simulink model "single_ph_controlled_rectifier_inductive_load"  (R2018a)
settings: Solver=ode23tb  StartTime=0  StopTime=2  MaxStep=1e-6  RelTol=1e-5
libraries: powerlib x10
settings Model: Creator=pranjal  LastModifiedBy=pranjal
settings HardwareCC: ProdBitPerLong=64  ProdHWDeviceType=AMD->x86-64 (Linux 64)

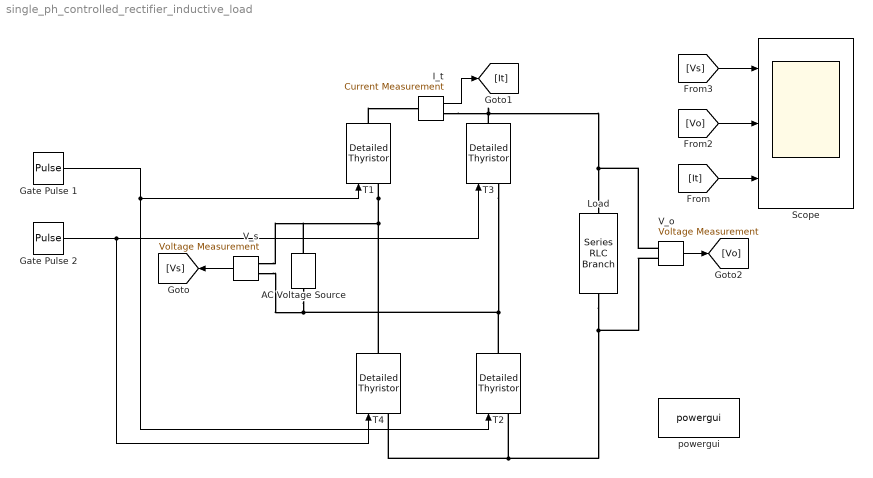
== system single_ph_controlled_rectifier_inductive_load ==
  AC Voltage Source : powerlib/Electrical Sources/AC Voltage Source  Amplitude=230*1.414  Phase=0  Frequency=50  SampleTime=0  Measurements=Voltage  BusType=swing  Pref=10e3  Qref=0  Qmin=-inf  Qmax=+inf
  Gate Pulse 1 : DiscretePulseGenerator  PulseType=Time based  Period=20e-3  PulseWidth=5  PhaseDelay=(30/360)*20e-3
  Gate Pulse 2 : DiscretePulseGenerator  PulseType=Time based  Period=20e-3  PulseWidth=5  PhaseDelay=((180+30)/360)*20e-3
  I_t : powerlib/Measurements/Current Measurement  PhasorSimulation=off  OutputType=Complex  PSBequivalent=0
  Load : powerlib/Elements/Series RLC Branch  LConnTagsString=__new0  RConnTagsString=__new0  BranchType=RL  Resistance=20  Inductance=5  SetiL0=off  InitialCurrent=0  Capacitance=1e-6  Setx0=off  InitialVoltage=0  Measurements=None
  Scope : Scope  NumInputPorts=3
  T{1..4} (4 alike) : powerlib/Power Electronics/Detailed Thyristor  Ron=0.001  Lon=1e-3  Vf=0.8  IL=0.1  Tq=100e-6  IC=0  Rs=500  Cs=250e-9  Measurements=off
      settings: SourceProductName=Simscape Power Systems  SourceProductBaseCode=PS
  V_o : powerlib/Measurements/Voltage Measurement  PhasorSimulation=off  OutputType=Complex  PSBequivalent=0
  V_s : powerlib/Measurements/Voltage Measurement  PhasorSimulation=off  OutputType=Complex  PSBequivalent=0
  powergui : powerlib/powergui  Priority=1  SimulationMode=Continuous  SampleTime=50e-6  frequency=60  Iterations=50  frequencyindice=50  Pbase=100e6  ErrMax=1e-4  UnitsV=kV  UnitsW=MW  buscounter=0  FunctionMessages=off  echomessages=off  EnableUseOfTLC=off  CurrentSourceSwitches=off  DisableSnubberDevices=off  DisableRonSwitches=off  DisableVfSwitches=off  DisplayEquations=off  SolverType=Tustin/Backward Euler (TBE)  Interpol=off  ExternalGateDelay=off  methode=off  Ts=100  x0status=blocks  SPID=on  SwTol=0  HookPort=off  RestoreLinks=warning  ResistiveCurrentMeasurement=off  Frange=[0:2:500]  Ylog=off  Xlog=on  ShowGrid=off  save=off  variable=ZData  structure=0  ZoomFFT=off  StartTime=0.0  cycles=1  DisplayStyle=1  fundamental=60  FreqAxis=off  MaxFrequency=1000  frequencyindicesteady=1  RmsSteady=1  display=off
  wires:
  V_s/1 -> [Vs]
  V_o/1 -> [Vo]
  [Vs] -> Scope/1
  Gate Pulse 2/1 -> T3/1, T4/1
  Gate Pulse 1/1 -> T2/1, T1/1
  I_t/1 -> [It]
  [Vo] -> Scope/2
  [It] -> Scope/3
  connections:
  I_t/RConn1 -- V_o/LConn1 -- Load/LConn1 -- T3/RConn1
  V_o/LConn2 -- T2/LConn1 -- T4/LConn1 -- Load/RConn1
  T1/LConn1 -- T4/RConn1 -- V_s/LConn1 -- AC Voltage Source/RConn1
  T3/LConn1 -- T2/RConn1 -- V_s/LConn2 -- AC Voltage Source/LConn1
  T1/RConn1 -- I_t/LConn1
